simulink model "s1"  (Simulink 2.00)
settings: Solver=ode45  StartTime=0.0  StopTime=tstop  MaxStep=5e-3  RelTol=5e-6  AbsTol=1e-6
values from neighbouring files (symbols this model uses):
  delto = delt    [M1.M]    (also in M3.M; M4.M = 0; M5.M)
  Domega = 0    [M4.M]    (also in SET1.M; SET3A.M; SET3B.M; SET3C.M)
  Ex_time = [0 tstop]    [M1.M]    (also in M5.M)
  Ex_value = [1 1]*Efo    [M1.M]    (also in M5.M)
  H = 0.5*J_rotor*wbasem*wbasem/Sbase    [M1.M]    (also in M3.M; M4.M = 0.3; SET1.M = 3.77; SET3A.M = 3)
  Psido = xls*(-Ido) + Psiado    [M1.M]    (also in M3.M; M4.M = Psiado; M5.M)
  Psifo = xplf*Ifo + Psiado    [M1.M]    (also in M3.M; M5.M = (xpr2c+xpr1c+xp1c)*Ifo + Psiado)
  Psikdo = Psiado    [M1.M]    (also in M3.M; M4.M)
  Psikqo = Psiaqo    [M1.M]    (also in M3.M; M4.M = 0)
  Psiqo = xls*(-Iqo) + Psiaqo    [M1.M]    (also in M3.M; M4.M = 0; M5.M)
  rpf = rpf/Zbase    [M1.M]    (also in M3.M; SET3A.M = 0.00112; SET3B.M = 0.00109)
  rpkd = rpkd/Zbase    [M1.M]    (also in M3.M; M4.M = 0.054)
  rpkq = rpkq/Zbase    [M1.M]    (also in M3.M; M4.M = 0.108)
  rs = rs/Zbase    [M1.M]    (also in M3.M; M4.M = 0.017; SET1.M = 0.0048; SET3A.M = 0.004)
  T2piby3 = 2*pi/3    (= 2.09439510239)    [M1.M]    (also in M5.M)
  thetaro = delto+thetaeo    [M1.M]    (also in M5.M)
  tmech_time = [0 tstop]    [M1.M]    (also in M4.M; M5.M)
  tmech_value = [1 1]*Tmech    [M1.M]    (also in M4.M = [-1 -1]*temo; M5.M)
  Vm_time = [0 tfstart tfstart (tfstart+tfault) (tfstart+tfault) tstop]    [M1.M]    (also in M5.M)
  Vm_value = [1 1 0 0 1 1]*Vm    [M1.M]    (also in M5.M)
  wb = wbase    [M1.M]    (also in M3.M; M4.M = 376.991118431; M5.M)
  xls = xls/Zbase    [M1.M]    (also in M3.M; M4.M = 0.065; SET1.M = 0.215; SET3A.M = 0.19)
  xmd = xmd/Zbase    [M1.M]    (also in M3.M; M4.M = 0.478; SET3A.M = 1.7; SET3B.M = 1.7)
  xMD = (1/xls + 1/xmd + 1/xplf + 1/xplkd)^(-1)    [M1.M]    (also in M3.M; M4.M = 0.0399162984447; M5.M = (1/xls + 1/xmd + bsum)^(-1))
  xMQ = (1/xls + 1/xmq + 1/xplkq)^(-1)    [M1.M]    (also in M3.M; M4.M = 0.0417714348384; M5.M = (1/xls + 1/xmq + 1/xplkq3 + 1/xplkq2 + 1/xplkq1)^(-1))
  xplf = xplf/Zbase    [M1.M]    (also in M3.M)
  xplkd = xplkd/Zbase    [M1.M]    (also in M3.M; M4.M = 0.132)
  xplkq = xplkq/Zbase    [M1.M]    (also in M3.M; M4.M = 0.132)
settings Model: SaveTime=off  SaveOutput=off  ConsistencyChecking=off

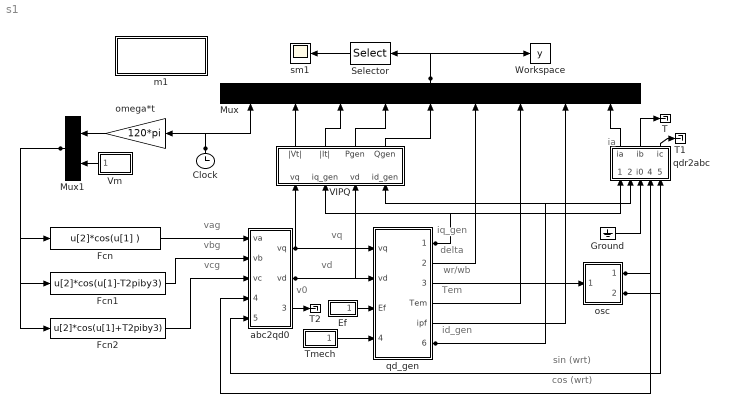
== system s1 ==
  note: iq_gen
  note: ia
  note: vag
  note: v0
  note: wr/wb
  note: id_gen
  note: delta
  note: Tem
  note: cos (wrt)
  note: sin (wrt)
  note: vq
  note: vd
  note: vbg
  note: vcg
  Clock : Clock
      settings: Orientation=up  DeleteFcn=simclock BlockIsBeingDestroyed  PostSaveFcn=simclock Save
  Ef : Subsystem  mask(Repeating table){rep_seq_t=Ex_time, rep_seq_y=Ex_value}
      mask prompts: rep_seq_t "Time values:"; rep_seq_y "Output values:"
      mask help: Repeating table.
      mask init:
      | period = max(rep_seq_t);
      mask Help: Repeats cycle given in table. Time values should be monotonically increasing.
      mask Display: plot([rep_seq_t,rep_seq_t+period,rep_seq_t+2*period,rep_seq_t(1)+3*period],[rep_seq_y,rep_seq_y,rep_seq_y,rep_seq_y(1)])
  Fcn : Fcn  Expr=u[2]*cos(u[1] )
  Fcn1 : Fcn  Expr=u[2]*cos(u[1]-T2piby3)
  Fcn2 : Fcn  Expr=u[2]*cos(u[1]+T2piby3)
  Ground : Ground
  m1 : Subsystem
      settings: OpenFcn=m1
      mask Type: Masked block of m1.m
      mask Help: Uses m1.m to initialize and plot
      mask Display: disp('Initialize\nand plot')
  Mux : Mux  Orientation=up  Inputs=9
  Mux1 : Mux  Orientation=left  Inputs=2
  Selector : Selector  Orientation=left  Elements=[2 4 5 6 7 9]  InputPortWidth=9
  T : Terminator
  T1 : Terminator
  T2 : Terminator
  Tmech : Subsystem  mask(Repeating table){rep_seq_t=tmech_time, rep_seq_y=tmech_value}
      mask prompts: rep_seq_t "Time values:"; rep_seq_y "Output values:"
      mask help: Repeating table.
      mask init:
      | period = max(rep_seq_t);
      mask Help: Repeats cycle given in table. Time values should be monotonically increasing.
      mask Display: plot([rep_seq_t,rep_seq_t+period,rep_seq_t+2*period,rep_seq_t(1)+3*period],[rep_seq_y,rep_seq_y,rep_seq_y,rep_seq_y(1)])
  VIPQ : Subsystem  Orientation=up
  Vm : Subsystem  Orientation=left  mask(Repeating table){rep_seq_t=Vm_time, rep_seq_y=Vm_value}
      mask prompts: rep_seq_t "Time values:"; rep_seq_y "Output values:"
      mask help: Repeating table.
      mask init:
      | period = max(rep_seq_t);
      mask Help: Repeats cycle given in table. Time values should be monotonically increasing.
      mask Display: plot([rep_seq_t,rep_seq_t+period,rep_seq_t+2*period,rep_seq_t(1)+3*period],[rep_seq_y,rep_seq_y,rep_seq_y,rep_seq_y(1)])
  Workspace : ToWorkspace  VariableName=y  SampleTime=0
      settings: Buffer=100000
  abc2qd0 : Subsystem
  omega*t : Gain  Orientation=left  Gain=120*pi
  osc : Subsystem
  qd_gen : Subsystem
  qdr2abc : Subsystem  Orientation=up
  sm1 : Scope
      settings: TickLabels=on  TimeRange=auto  YMin=-2  YMax=2  SaveToWorkspace=off  SaveName=ScopeData  LimitMaxRows=off
  wires:
  Vm/1(out_1) -> Mux1/2
  Ef/1(out_1) -> qd_gen/3(Ef)
  Selector/1 -> sm1/1
  Mux/1 -> Selector/1, Workspace/1
  Ground/1 -> qdr2abc/3(i0)
  qdr2abc/3(ic) -> T1/1
  qdr2abc/2(ib) -> T/1
  abc2qd0/3(vd0) -> T2/1
  VIPQ/2(|It|) -> Mux/3
  VIPQ/3(Pgen) -> Mux/4
  VIPQ/4(Qgen) -> Mux/5
  qd_gen/2(delta) -> Mux/6
  qd_gen/4(Tem) -> Mux/7
  qd_gen/5(ipf) -> Mux/8
  qdr2abc/1(ia) -> Mux/9
  Fcn2/1 -> abc2qd0/3(vc)
  Fcn1/1 -> abc2qd0/2(vb)
  Fcn/1 -> abc2qd0/1(va)
  Mux1/1 -> Fcn2/1, Fcn1/1, Fcn/1
  omega*t/1 -> Mux1/1
  Clock/1 -> omega*t/1, Mux/1
  abc2qd0/2(vd) -> VIPQ/3(vd), qd_gen/2(vd)
  VIPQ/1(|Vt|) -> Mux/2
  Tmech/1(out_1) -> qd_gen/4(Tmech)
  qd_gen/6(id_gen) -> VIPQ/4(id_gen), qdr2abc/2(-id)
  qd_gen/3(wr/wb) -> osc/1(wr/wb)
  qd_gen/1(iq_gen) -> VIPQ/2(iq_gen), qdr2abc/1(-iq)
  abc2qd0/1(vq) -> VIPQ/1(vq), qd_gen/1(vq)
  osc/2(sin_thetar) -> abc2qd0/5(sin_thetar), qdr2abc/5(sin_thetar)
  osc/1(cos_thetar) -> abc2qd0/4(cos_thetar), qdr2abc/4(cos_thetar)

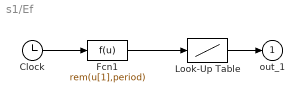
== system s1/Ef ==
  Clock : Clock
      settings: DeleteFcn=simclock BlockIsBeingDestroyed  PostSaveFcn=simclock Save
  Fcn1 : Fcn  Expr=rem(u[1],period)
  Look-Up Table : Lookup  InputValues=rep_seq_t  OutputValues=rep_seq_y
  out_1 : Outport  Port=1  InitialOutput=0
  wires:
  Fcn1/1 -> Look-Up Table/1
  Clock/1 -> Fcn1/1
  Look-Up Table/1 -> out_1/1

== system s1/m1 ==
  note: Masked block of m1.m to
      | initialize and print results

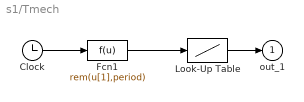
== system s1/Tmech ==
  Clock : Clock
      settings: DeleteFcn=simclock BlockIsBeingDestroyed  PostSaveFcn=simclock Save
  Fcn1 : Fcn  Expr=rem(u[1],period)
  Look-Up Table : Lookup  InputValues=rep_seq_t  OutputValues=rep_seq_y
  out_1 : Outport  Port=1  InitialOutput=0
  wires:
  Fcn1/1 -> Look-Up Table/1
  Clock/1 -> Fcn1/1
  Look-Up Table/1 -> out_1/1

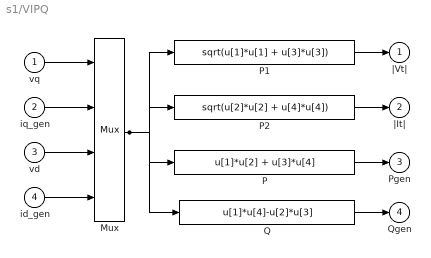
== system s1/VIPQ ==
  vq : Inport  Port=1  PortWidth=-1  SampleTime=-1
  iq_gen : Inport  Port=2  PortWidth=-1  SampleTime=-1
  vd : Inport  Port=3  PortWidth=-1  SampleTime=-1
  id_gen : Inport  Port=4  PortWidth=-1  SampleTime=-1
  Mux : Mux  Inputs=4
  P : Fcn  Expr=u[1]*u[2] + u[3]*u[4]
  P1 : Fcn  Expr=sqrt(u[1]*u[1] + u[3]*u[3])
  P2 : Fcn  Expr=sqrt(u[2]*u[2] + u[4]*u[4])
  Q : Fcn  Expr=u[1]*u[4]-u[2]*u[3]
  |Vt| : Outport  Port=1  InitialOutput=0
  |It| : Outport  Port=2  InitialOutput=0
  Pgen : Outport  Port=3  InitialOutput=0
  Qgen : Outport  Port=4  InitialOutput=0
  wires:
  P2/1 -> |It|/1
  P1/1 -> |Vt|/1
  Mux/1 -> P2/1, P1/1, Q/1, P/1
  Q/1 -> Qgen/1
  P/1 -> Pgen/1
  id_gen/1 -> Mux/4
  vd/1 -> Mux/3
  iq_gen/1 -> Mux/2
  vq/1 -> Mux/1

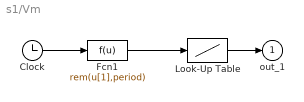
== system s1/Vm ==
  Clock : Clock
      settings: DeleteFcn=simclock BlockIsBeingDestroyed  PostSaveFcn=simclock Save
  Fcn1 : Fcn  Expr=rem(u[1],period)
  Look-Up Table : Lookup  InputValues=rep_seq_t  OutputValues=rep_seq_y
  out_1 : Outport  Port=1  InitialOutput=0
  wires:
  Fcn1/1 -> Look-Up Table/1
  Clock/1 -> Fcn1/1
  Look-Up Table/1 -> out_1/1

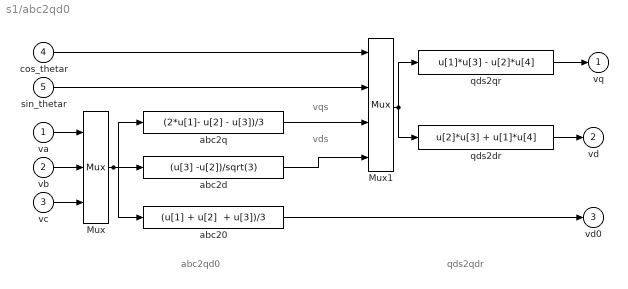
== system s1/abc2qd0 ==
  note: vqs
  note: qds2qdr
  note: abc2qd0
  note: vds
  va : Inport  Port=1  PortWidth=-1  SampleTime=-1
  vb : Inport  Port=2  PortWidth=-1  SampleTime=-1
  vc : Inport  Port=3  PortWidth=-1  SampleTime=-1
  cos_thetar : Inport  Port=4  PortWidth=-1  SampleTime=-1
  sin_thetar : Inport  Port=5  PortWidth=-1  SampleTime=-1
  Mux : Mux  Inputs=3
  Mux1 : Mux  Inputs=4
  abc20 : Fcn  Expr="(u[1] + u[2]  + u[3])/3"
  abc2d : Fcn  Expr=(u[3] -u[2])/sqrt(3)
  abc2q : Fcn  Expr=(2*u[1]- u[2] - u[3])/3
  qds2dr : Fcn  Expr=u[2]*u[3] + u[1]*u[4]
  qds2qr : Fcn  Expr=u[1]*u[3] - u[2]*u[4]
  vq : Outport  Port=1  InitialOutput=0
  vd : Outport  Port=2  InitialOutput=0
  vd0 : Outport  Port=3  InitialOutput=0
  wires:
  abc20/1 -> vd0/1
  abc2d/1 -> Mux1/4
  abc2q/1 -> Mux1/3
  sin_thetar/1 -> Mux1/2
  cos_thetar/1 -> Mux1/1
  qds2dr/1 -> vd/1
  qds2qr/1 -> vq/1
  vc/1 -> Mux/3
  vb/1 -> Mux/2
  va/1 -> Mux/1
  Mux1/1 -> qds2dr/1, qds2qr/1
  Mux/1 -> abc20/1, abc2d/1, abc2q/1

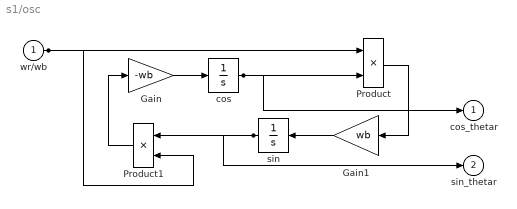
== system s1/osc ==
  wr/wb : Inport  Port=1  PortWidth=-1  SampleTime=-1
  Gain : Gain  Gain=-wb
  Gain1 : Gain  Orientation=left  Gain=wb
  Product : Product  Inputs=2
  Product1 : Product  Orientation=left  Inputs=2
  cos : Integrator  ExternalReset=none  InitialConditionSource=internal  InitialCondition=cos(thetaro)  LimitOutput=off  UpperSaturationLimit=inf  LowerSaturationLimit=-inf  ShowSaturationPort=off  ShowStatePort=off  AbsoluteTolerance=auto
  sin : Integrator  Orientation=left  ExternalReset=none  InitialConditionSource=internal  InitialCondition=sin(thetaro)  LimitOutput=off  UpperSaturationLimit=inf  LowerSaturationLimit=-inf  ShowSaturationPort=off  ShowStatePort=off  AbsoluteTolerance=auto
  cos_thetar : Outport  Port=1  InitialOutput=0
  sin_thetar : Outport  Port=2  InitialOutput=0
  wires:
  sin/1 -> sin_thetar/1, Product1/1
  wr/wb/1 -> Product1/2, Product/1
  Gain1/1 -> sin/1
  Product1/1 -> Gain/1
  Gain/1 -> cos/1
  cos/1 -> Product/2, cos_thetar/1
  Product/1 -> Gain1/1

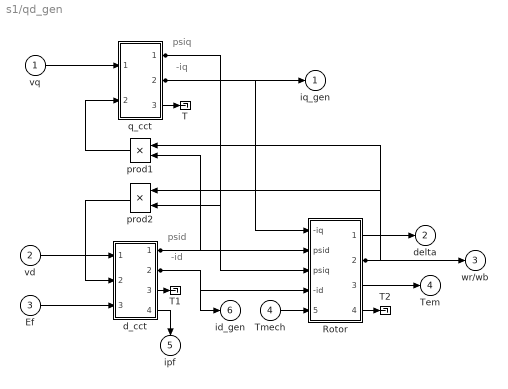
== system s1/qd_gen ==
  note: psiq
  note: psid
  note: -id
  note: -iq
  vq : Inport  Port=1  PortWidth=-1  SampleTime=-1
  vd : Inport  Port=2  PortWidth=-1  SampleTime=-1
  Ef : Inport  Port=3  PortWidth=-1  SampleTime=-1
  Tmech : Inport  Port=4  PortWidth=-1  SampleTime=-1
  Rotor : Subsystem
  T : Terminator
  T1 : Terminator
  T2 : Terminator
  d_cct : Subsystem
  prod1 : Product  Orientation=left  Inputs=2
  prod2 : Product  Orientation=left  Inputs=2
  q_cct : Subsystem
  iq_gen : Outport  Port=1  InitialOutput=0
  delta : Outport  Port=2  InitialOutput=0
  wr/wb : Outport  Port=3  InitialOutput=0
  Tem : Outport  Port=4  InitialOutput=0
  ipf : Outport  Orientation=down  Port=5  InitialOutput=0
  id_gen : Outport  Port=6  InitialOutput=0
  wires:
  Rotor/4((wr-we)/wb) -> T2/1
  d_cct/3(Out_psimd) -> T1/1
  q_cct/3(Out_psimq) -> T/1
  d_cct/4(Out_ipf) -> ipf/1
  prod2/1 -> d_cct/2(In_wrpsiq)
  vd/1 -> d_cct/1(In_vd)
  Ef/1 -> d_cct/3(In_Ef)
  q_cct/1(Out_psiq) -> prod2/2, Rotor/3(psiq)
  Rotor/2("wr/wb ") -> prod2/1, prod1/1, wr/wb/1
  d_cct/1(Out_psid) -> prod1/2, Rotor/2("psid ")
  vq/1 -> q_cct/1(In_vq)
  prod1/1 -> q_cct/2(In_wrpsid)
  d_cct/2(Out_-id) -> id_gen/1, Rotor/4(-id)
  Rotor/3(Tem) -> Tem/1
  Rotor/1(delta) -> delta/1
  q_cct/2(Out_-iq) -> iq_gen/1, Rotor/1(-iq)
  Tmech/1 -> Rotor/5(Tmech)

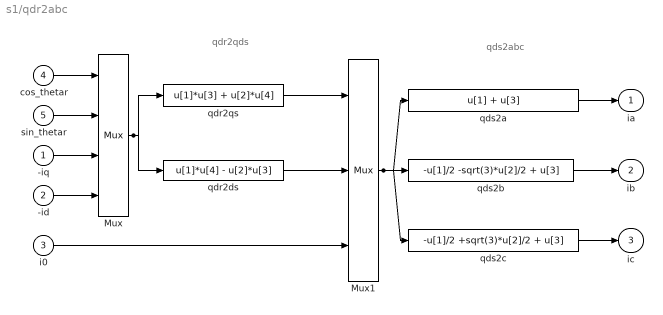
== system s1/qdr2abc ==
  note: qds2abc
  note: qdr2qds
  -iq : Inport  Port=1  PortWidth=-1  SampleTime=-1
  -id : Inport  Port=2  PortWidth=-1  SampleTime=-1
  i0 : Inport  Port=3  PortWidth=-1  SampleTime=-1
  cos_thetar : Inport  Port=4  PortWidth=-1  SampleTime=-1
  sin_thetar : Inport  Port=5  PortWidth=-1  SampleTime=-1
  Mux : Mux  Inputs=4
  Mux1 : Mux  Inputs=3
  qdr2ds : Fcn  Expr=u[1]*u[4] - u[2]*u[3]
  qdr2qs : Fcn  Expr=u[1]*u[3] + u[2]*u[4]
  qds2a : Fcn  Expr=u[1] + u[3]
  qds2b : Fcn  Expr=-u[1]/2 -sqrt(3)*u[2]/2 + u[3]
  qds2c : Fcn  Expr=-u[1]/2 +sqrt(3)*u[2]/2 + u[3]
  ia : Outport  Port=1  InitialOutput=0
  ib : Outport  Port=2  InitialOutput=0
  ic : Outport  Port=3  InitialOutput=0
  wires:
  qds2c/1 -> ic/1
  qds2b/1 -> ib/1
  qds2a/1 -> ia/1
  Mux1/1 -> qds2c/1, qds2a/1, qds2b/1
  i0/1 -> Mux1/3
  qdr2ds/1 -> Mux1/2
  qdr2qs/1 -> Mux1/1
  Mux/1 -> qdr2ds/1, qdr2qs/1
  -id/1 -> Mux/4
  -iq/1 -> Mux/3
  sin_thetar/1 -> Mux/2
  cos_thetar/1 -> Mux/1

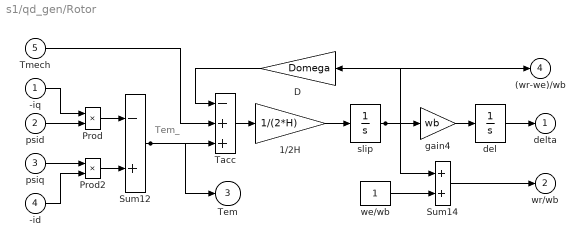
== system s1/qd_gen/Rotor ==
  note: Tem_
  -iq : Inport  Port=1  PortWidth=-1  SampleTime=-1
  "psid " : Inport  Port=2  PortWidth=-1  SampleTime=-1
  psiq : Inport  Port=3  PortWidth=-1  SampleTime=-1
  -id : Inport  Port=4  PortWidth=-1  SampleTime=-1
  Tmech : Inport  Port=5  PortWidth=-1  SampleTime=-1
  1/2H : Gain  Gain=1/(2*H)
  D : Gain  Orientation=left  Gain=Domega
  Prod : Product  Inputs=2
  Prod2 : Product  Inputs=2
  Sum12 : Sum  Inputs=-+
  Sum14 : Sum  Inputs=++
  Tacc : Sum  Inputs=-++
  del : Integrator  ExternalReset=none  InitialConditionSource=internal  InitialCondition=delto  LimitOutput=off  UpperSaturationLimit=inf  LowerSaturationLimit=-inf  ShowSaturationPort=off  ShowStatePort=off  AbsoluteTolerance=auto
  gain4 : Gain  Gain=wb
  slip : Integrator  ExternalReset=none  InitialConditionSource=internal  InitialCondition=0  LimitOutput=off  UpperSaturationLimit=inf  LowerSaturationLimit=-inf  ShowSaturationPort=off  ShowStatePort=off  AbsoluteTolerance=auto
  we/wb : Constant  Value=1
  delta : Outport  Port=1  InitialOutput=0
  "wr/wb " : Outport  Port=2  InitialOutput=0
  Tem : Outport  Port=3  InitialOutput=0
  (wr-we)/wb : Outport  Port=4  InitialOutput=0
  wires:
  Tmech/1 -> Tacc/2
  slip/1 -> D/1, (wr-we)/wb/1, Sum14/1, gain4/1
  Sum12/1 -> Tem/1, Tacc/3
  Sum14/1 -> "wr/wb "/1
  -id/1 -> Prod2/2
  psiq/1 -> Prod2/1
  del/1 -> delta/1
  "psid "/1 -> Prod/2
  -iq/1 -> Prod/1
  Prod/1 -> Sum12/1
  Tacc/1 -> 1/2H/1
  we/wb/1 -> Sum14/2
  1/2H/1 -> slip/1
  Prod2/1 -> Sum12/2
  gain4/1 -> del/1
  D/1 -> Tacc/1

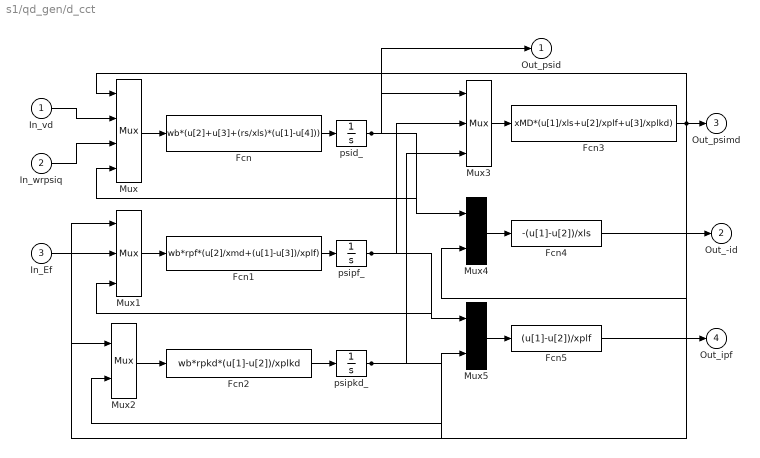
== system s1/qd_gen/d_cct ==
  In_vd : Inport  Port=1  PortWidth=-1  SampleTime=-1
  In_wrpsiq : Inport  Port=2  PortWidth=-1  SampleTime=-1
  In_Ef : Inport  Port=3  PortWidth=-1  SampleTime=-1
  Fcn : Fcn  Expr=wb*(u[2]+u[3]+(rs/xls)*(u[1]-u[4]))
  Fcn1 : Fcn  Expr=wb*rpf*(u[2]/xmd+(u[1]-u[3])/xplf)
  Fcn2 : Fcn  Expr=wb*rpkd*(u[1]-u[2])/xplkd
  Fcn3 : Fcn  Expr=xMD*(u[1]/xls+u[2]/xplf+u[3]/xplkd)
  Fcn4 : Fcn  Expr=-(u[1]-u[2])/xls
  Fcn5 : Fcn  Expr=(u[1]-u[2])/xplf
  Mux : Mux  Inputs=4
  Mux1 : Mux  Inputs=3
  Mux2 : Mux  Inputs=2
  Mux3 : Mux  Inputs=3
  Mux4 : Mux  Inputs=2
  Mux5 : Mux  Inputs=2
  psid_ : Integrator  ExternalReset=none  InitialConditionSource=internal  InitialCondition=Psido  LimitOutput=off  UpperSaturationLimit=inf  LowerSaturationLimit=-inf  ShowSaturationPort=off  ShowStatePort=off  AbsoluteTolerance=auto
  psipf_ : Integrator  ExternalReset=none  InitialConditionSource=internal  InitialCondition=Psifo  LimitOutput=off  UpperSaturationLimit=inf  LowerSaturationLimit=-inf  ShowSaturationPort=off  ShowStatePort=off  AbsoluteTolerance=auto
  psipkd_ : Integrator  ExternalReset=none  InitialConditionSource=internal  InitialCondition=Psikdo  LimitOutput=off  UpperSaturationLimit=inf  LowerSaturationLimit=-inf  ShowSaturationPort=off  ShowStatePort=off  AbsoluteTolerance=auto
  Out_psid : Outport  Port=1  InitialOutput=0
  Out_-id : Outport  Port=2  InitialOutput=0
  Out_psimd : Outport  Port=3  InitialOutput=0
  Out_ipf : Outport  Port=4  InitialOutput=0
  wires:
  Mux2/1 -> Fcn2/1
  In_Ef/1 -> Mux1/2
  Mux1/1 -> Fcn1/1
  Mux/1 -> Fcn/1
  In_vd/1 -> Mux/2
  In_wrpsiq/1 -> Mux/3
  Fcn5/1 -> Out_ipf/1
  Fcn4/1 -> Out_-id/1
  Fcn3/1 -> Out_psimd/1, Mux/1, Mux1/1, Mux2/1, Mux4/2, Mux5/2
  Mux5/1 -> Fcn5/1
  Mux4/1 -> Fcn4/1
  Mux3/1 -> Fcn3/1
  psipkd_/1 -> Mux3/3, Mux2/2
  psipf_/1 -> Mux5/1, Mux3/2, Mux1/3
  psid_/1 -> Out_psid/1, Mux4/1, Mux3/1, Mux/4
  Fcn2/1 -> psipkd_/1
  Fcn1/1 -> psipf_/1
  Fcn/1 -> psid_/1

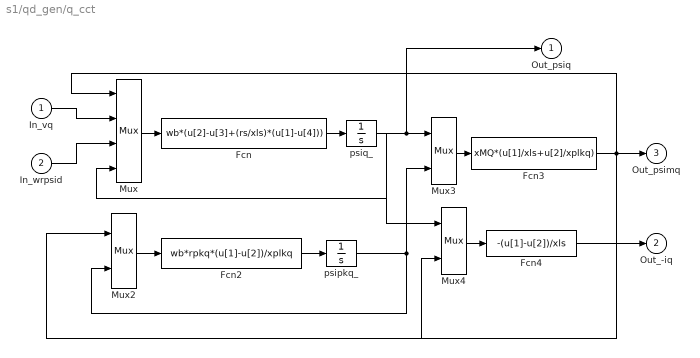
== system s1/qd_gen/q_cct ==
  In_vq : Inport  Port=1  PortWidth=-1  SampleTime=-1
  In_wrpsid : Inport  Port=2  PortWidth=-1  SampleTime=-1
  Fcn : Fcn  Expr=wb*(u[2]-u[3]+(rs/xls)*(u[1]-u[4]))
  Fcn2 : Fcn  Expr=wb*rpkq*(u[1]-u[2])/xplkq
  Fcn3 : Fcn  Expr=xMQ*(u[1]/xls+u[2]/xplkq)
  Fcn4 : Fcn  Expr=-(u[1]-u[2])/xls
  Mux : Mux  Inputs=4
  Mux2 : Mux  Inputs=2
  Mux3 : Mux  Inputs=2
  Mux4 : Mux  Inputs=2
  psipkq_ : Integrator  ExternalReset=none  InitialConditionSource=internal  InitialCondition=Psikqo  LimitOutput=off  UpperSaturationLimit=inf  LowerSaturationLimit=-inf  ShowSaturationPort=off  ShowStatePort=off  AbsoluteTolerance=auto
  psiq_ : Integrator  ExternalReset=none  InitialConditionSource=internal  InitialCondition=Psiqo  LimitOutput=off  UpperSaturationLimit=inf  LowerSaturationLimit=-inf  ShowSaturationPort=off  ShowStatePort=off  AbsoluteTolerance=auto
  Out_psiq : Outport  Port=1  InitialOutput=0
  Out_-iq : Outport  Port=2  InitialOutput=0
  Out_psimq : Outport  Port=3  InitialOutput=0
  wires:
  Fcn4/1 -> Out_-iq/1
  Fcn3/1 -> Out_psimq/1, Mux/1, Mux2/1, Mux4/2
  Mux4/1 -> Fcn4/1
  Mux3/1 -> Fcn3/1
  psipkq_/1 -> Mux3/2, Mux2/2
  psiq_/1 -> Out_psiq/1, Mux4/1, Mux3/1, Mux/4
  Fcn2/1 -> psipkq_/1
  Mux2/1 -> Fcn2/1
  Fcn/1 -> psiq_/1
  Mux/1 -> Fcn/1
  In_vq/1 -> Mux/2
  In_wrpsid/1 -> Mux/3
